simulink model "FamlyLStateCtrl"  (R2018b)
settings: Solver=FixedStepDiscrete  StartTime=0.0  StopTime=10.0  FixedStep=0.01  RelTol=1e-3
libraries: StateCtrlLib x1
settings Model: Creator=sn2xws  LastModifiedBy=sn2xws
settings DataIOCC: SaveFormat=StructureWithTime
settings OptimizationCC: DefaultParameterBehavior=Inlined  EnhancedBackFolding=on  PassReuseOutputArgsAs=Individual arguments  ZeroExternalMemoryAtStartup=off  ZeroInternalMemoryAtStartup=off  OptimizeBlockOrder=speed  DifferentSizesBufferReuse=on  OptimizationCustomize=off
settings DebuggingCC: ParameterTunabilityLossMsg=error
settings ModelReferenceCC: ModelReferenceNumInstancesAllowed=Single
settings SFSimCC: MATLABDynamicMemAlloc=off
settings RTWCC: SystemTargetFile=autosar.tlc  GenCodeOnly=on  TemplateMakefile=ert_default_tmf  Description=AUTOSAR  GenerateReport=on  IncludeHyperlinkInReport=on  LaunchReport=on  GenerateTraceInfo=on  GenerateTraceReport=on  GenerateTraceReportSl=on  GenerateTraceReportSf=on  GenerateTraceReportEml=on
settings CodeAppCC: ForceParamTrailComments=on  IgnoreCustomStorageClasses=off  OperatorAnnotations=on  SimulinkDataObjDesc=on  SFDataObjDesc=on  InsertBlockDesc=on
settings STFCustomTargetCC: TargetLangStandard=C99 (ISO)  MultiwordLength=256  ParMdlRefBuildCompliant=on  CompOptLevelCompliant=on  IncludeMdlTerminateFcn=off  CombineOutputUpdateFcns=on  SuppressErrorStatus=on  ERTCustomFileBanners=on  SupportNonFinite=off  SupportComplex=off  SupportContinuousTime=off  SupportNonInlinedSFcns=off  RemoveResetFunc=on  MATLABClassNameForMDSCustomization=Simulink.SoftwareTarget.ERTCustomization  AutosarCompliant=on  UseToolchainInfoCompliant=on  LookupTableObjectStructAxisOrder=2,1,3,4,...  LUTObjectStructOrderEvenSpacing=Size,Table,Breakpoints  SystemTargetFile=autosar.tlc
settings ERTTargetCC: TargetLangStandard=C99 (ISO)  ConcurrentExecutionCompliant=off  IncludeMdlTerminateFcn=off  SuppressErrorStatus=on  SupportNonFinite=off  SupportComplex=off  ModelStepFunctionPrototypeControlCompliant=off  CPPClassGenCompliant=off  AutosarCompliant=on  LookupTableObjectStructAxisOrder=2,1,3,4,...  LUTObjectStructOrderEvenSpacing=Size,Table,Breakpoints  InlinedParameterPlacement=NonHierarchical  ERTCustomFileTemplate=example_file_process.tlc

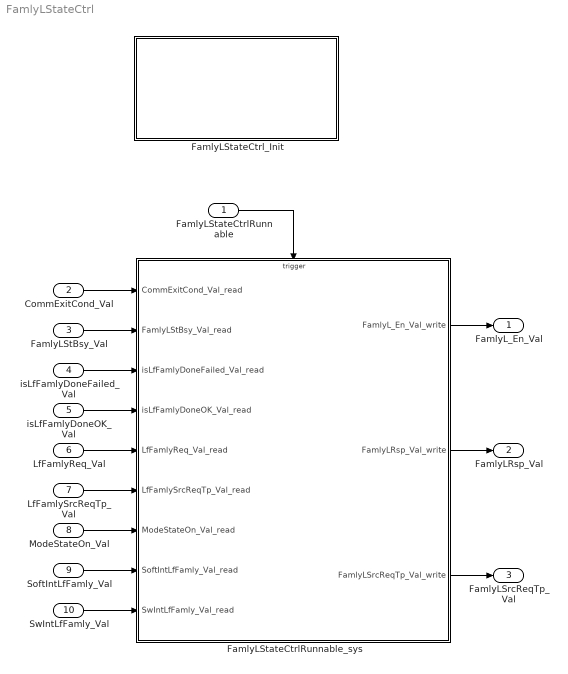
== system FamlyLStateCtrl ==
  FamlyLStateCtrlRunnable : Inport  SampleTime=0.01  OutputFunctionCall=on
  CommExitCond_Val : Inport  Port=2  OutDataTypeStr=boolean  PortDimensions=1
  FamlyLStBsy_Val : Inport  Port=3  OutDataTypeStr=boolean  PortDimensions=1
  isLfFamlyDoneFailed_Val : Inport  Port=4  OutDataTypeStr=boolean  PortDimensions=1
  isLfFamlyDoneOK_Val : Inport  Port=5  OutDataTypeStr=boolean  PortDimensions=1
  LfFamlyReq_Val : Inport  Port=6  OutDataTypeStr=boolean  PortDimensions=1
  LfFamlySrcReqTp_Val : Inport  Port=7  OutDataTypeStr=Enum: SrcReqTp1  PortDimensions=1
  ModeStateOn_Val : Inport  Port=8  OutDataTypeStr=boolean  PortDimensions=1
  SoftIntLfFamly_Val : Inport  Port=9  OutDataTypeStr=IntEnable  PortDimensions=1
  SwIntLfFamly_Val : Inport  Port=10  OutDataTypeStr=IntEnable  PortDimensions=1
  FamlyLStateCtrlRunnable_sys : Subsystem
  FamlyLStateCtrl_Init : Subsystem
  FamlyL_En_Val : Outport  OutDataTypeStr=boolean  PortDimensions=1
  FamlyLRsp_Val : Outport  Port=2  OutDataTypeStr=Enum: MdRspLocal1  PortDimensions=1
  FamlyLSrcReqTp_Val : Outport  Port=3  OutDataTypeStr=Enum: SrcReqTp1  PortDimensions=1
  wires:
  CommExitCond_Val/1 -> FamlyLStateCtrlRunnable_sys/1(CommExitCond_Val_read)
  FamlyLStBsy_Val/1 -> FamlyLStateCtrlRunnable_sys/2(FamlyLStBsy_Val_read)
  isLfFamlyDoneFailed_Val/1 -> FamlyLStateCtrlRunnable_sys/3(isLfFamlyDoneFailed_Val_read)
  isLfFamlyDoneOK_Val/1 -> FamlyLStateCtrlRunnable_sys/4(isLfFamlyDoneOK_Val_read)
  LfFamlyReq_Val/1 -> FamlyLStateCtrlRunnable_sys/5(LfFamlyReq_Val_read)
  LfFamlySrcReqTp_Val/1 -> FamlyLStateCtrlRunnable_sys/6(LfFamlySrcReqTp_Val_read)
  ModeStateOn_Val/1 -> FamlyLStateCtrlRunnable_sys/7(ModeStateOn_Val_read)
  SoftIntLfFamly_Val/1 -> FamlyLStateCtrlRunnable_sys/8(SoftIntLfFamly_Val_read)
  SwIntLfFamly_Val/1 -> FamlyLStateCtrlRunnable_sys/9(SwIntLfFamly_Val_read)
  FamlyLStateCtrlRunnable_sys/1(FamlyL_En_Val_write) -> FamlyL_En_Val/1
  FamlyLStateCtrlRunnable_sys/2(FamlyLRsp_Val_write) -> FamlyLRsp_Val/1
  FamlyLStateCtrlRunnable_sys/3(FamlyLSrcReqTp_Val_write) -> FamlyLSrcReqTp_Val/1
  FamlyLStateCtrlRunnable/1 -> FamlyLStateCtrlRunnable_sys/Trigger

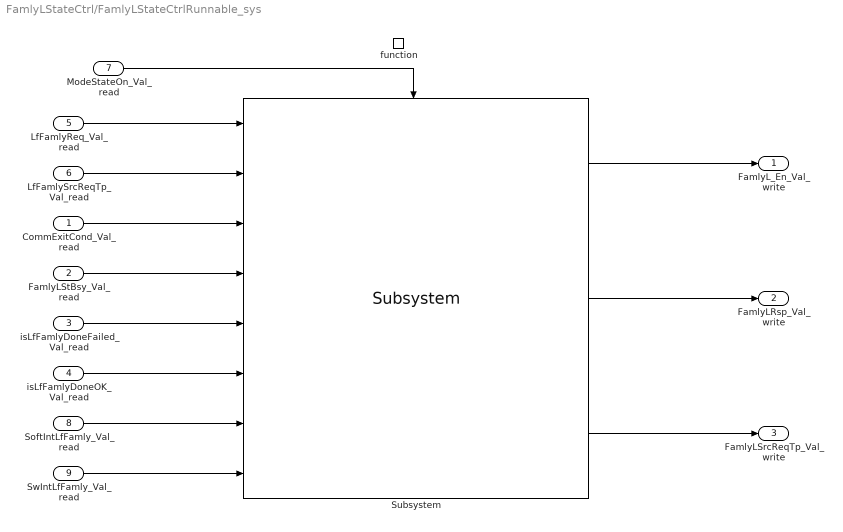
== system FamlyLStateCtrl/FamlyLStateCtrlRunnable_sys ==
  CommExitCond_Val_read : Inport
  FamlyLStBsy_Val_read : Inport  Port=2
  isLfFamlyDoneFailed_Val_read : Inport  Port=3
  isLfFamlyDoneOK_Val_read : Inport  Port=4
  LfFamlyReq_Val_read : Inport  Port=5
  LfFamlySrcReqTp_Val_read : Inport  Port=6
  ModeStateOn_Val_read : Inport  Port=7
  SoftIntLfFamly_Val_read : Inport  Port=8  OutDataTypeStr=IntEnable
  SwIntLfFamly_Val_read : Inport  Port=9  OutDataTypeStr=IntEnable
  function : TriggerPort  TriggerType=function-call  VariantControl=(inherit)  SampleTimeType=periodic  SampleTime=-1
  Subsystem : StateCtrlLib/Subsystem  SystemSampleTime=-1
  FamlyL_En_Val_write : Outport
      settings: EnsureOutportIsVirtual=on
  FamlyLRsp_Val_write : Outport  Port=2
      settings: EnsureOutportIsVirtual=on
  FamlyLSrcReqTp_Val_write : Outport  Port=3
      settings: EnsureOutportIsVirtual=on
  wires:
  CommExitCond_Val_read/1 -> Subsystem/3
  FamlyLStBsy_Val_read/1 -> Subsystem/4
  isLfFamlyDoneFailed_Val_read/1 -> Subsystem/5
  isLfFamlyDoneOK_Val_read/1 -> Subsystem/6
  LfFamlyReq_Val_read/1 -> Subsystem/1
  LfFamlySrcReqTp_Val_read/1 -> Subsystem/2
  ModeStateOn_Val_read/1 -> Subsystem/Enable
  SoftIntLfFamly_Val_read/1 -> Subsystem/7
  SwIntLfFamly_Val_read/1 -> Subsystem/8
  Subsystem/1 -> FamlyL_En_Val_write/1
  Subsystem/2 -> FamlyLRsp_Val_write/1
  Subsystem/3 -> FamlyLSrcReqTp_Val_write/1

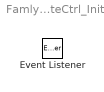
== system FamlyLStateCtrl/FamlyLStateCtrl_Init ==
  Event Listener : EventListener  EventName=reset
